simulink model "Aufgabe2b"  (R2020a)
settings: Solver=ode45  StartTime=0.0  StopTime=10.0  RelTol=1e-9
undefined symbols (not defined in the file or in its folder): A, A0, A1, B, B0, B1, C, D, x0
settings Model: Creator=Ravi Plenzdorf  LastModifiedBy=Ravi Plenzdorf
settings DataIOCC: ReturnWorkspaceOutputs=off

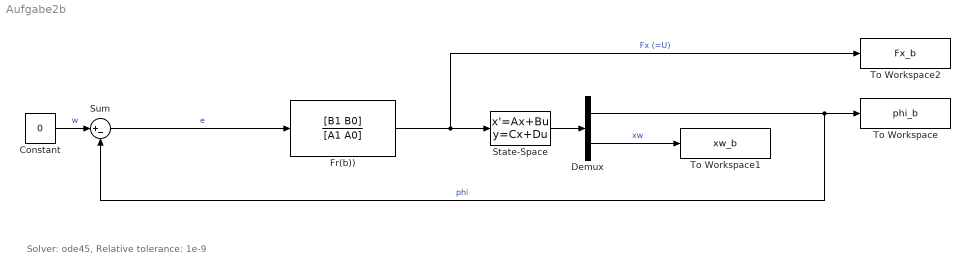
== system Aufgabe2b ==
  note: Solver: ode45, Relative tolerance: 1e-9
  Constant : Constant  Value=0
  Demux : Demux  Outputs=2
  Fr(b)) : TransferFcn  Numerator=[B1 B0]  Denominator=[A1 A0]
  State-Space : StateSpace  A=A  B=B  C=C  D=D  InitialCondition=x0
  Sum : Sum  Inputs=|+-
  To Workspace : ToWorkspace  VariableName=phi_b  SaveFormat=Timeseries  SampleTime=-1
  To Workspace1 : ToWorkspace  VariableName=xw_b  SaveFormat=Timeseries  SampleTime=-1
  To Workspace2 : ToWorkspace  VariableName=Fx_b  SaveFormat=Timeseries  SampleTime=-1
  wires:
  Fr(b))/1 -> State-Space/1, To Workspace2/1  "Fx (=U)"
  Demux/2 -> To Workspace1/1  "xw"
  State-Space/1 -> Demux/1
  Demux/1 -> To Workspace/1, Sum/2  "phi"
  Constant/1 -> Sum/1  "w"
  Sum/1 -> Fr(b))/1  "e"
